simulink model "pitch_control_loop"  (R2025a)
settings: Solver=ode4  StartTime=0.0  StopTime=10.0  FixedStep=0.05  RelTol=1e-3
undefined symbols (not defined in the file or in its folder): pid_damping_b, pitch_inertia
settings Model: Creator=saipr  LastModifiedBy=saipr
settings OptimizationCC: DefaultParameterBehavior=Inlined  EnhancedBackFolding=on  PassReuseOutputArgsAs=Individual arguments  ZeroExternalMemoryAtStartup=off  ZeroInternalMemoryAtStartup=off  OptimizeBlockOrder=speed  DifferentSizesBufferReuse=on  OptimizationCustomize=off  EfficientTunableParamExpr=on
settings DebuggingCC: ParameterTunabilityLossMsg=error
settings SFSimCC: MATLABDynamicMemAlloc=off
settings RTWCC: SystemTargetFile=ert.tlc  TemplateMakefile=ert_default_tmf  GenerateReport=on  GenerateTraceInfo=on  GenerateTraceReport=on  Description=Embedded Coder
settings CodeAppCC: ForceParamTrailComments=on  IgnoreCustomStorageClasses=off  OperatorAnnotations=on  SimulinkDataObjDesc=on  SFDataObjDesc=on  InsertBlockDesc=on
settings ERTTargetCC: ExtModeTransport=0.0  ExtModeStaticAlloc=off  ExtModeMexFile=ext_comm  ExtModeIntrfLevel=Level1  ERTCustomFileTemplate=example_file_process.tlc  TargetLangStandard=C99 (ISO)  GenerateSampleERTMain=on  SupportContinuousTime=on

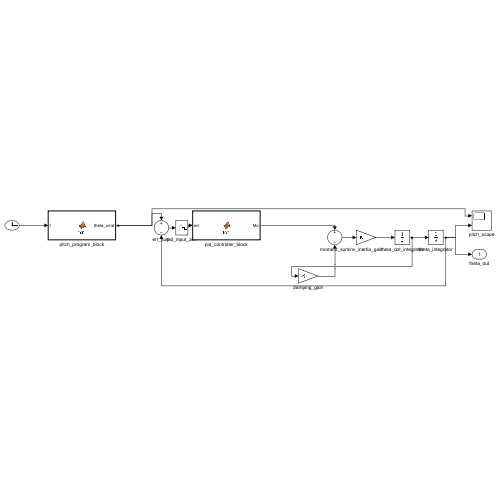
[thumbnail: Simulink's stored preview of the top-level diagram]
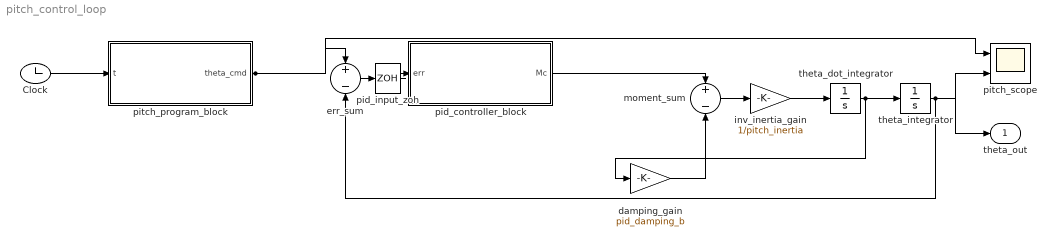
== system pitch_control_loop ==
  Clock : Clock
  damping_gain : Gain  Gain=pid_damping_b
  err_sum : Sum  Inputs=+-
  inv_inertia_gain : Gain  Gain=1/pitch_inertia
  moment_sum : Sum  Inputs=+-
  pid_controller_block : MATLAB Function  TreatAsAtomicUnit=on
  pid_input_zoh : ZeroOrderHold  SampleTime=0.05
  pitch_program_block : MATLAB Function  TreatAsAtomicUnit=on
  pitch_scope : Scope  NumInputPorts=2
  theta_dot_integrator : Integrator
  theta_integrator : Integrator
  theta_out : Outport
  wires:
  Clock/1 -> pitch_program_block/1(t)
  pitch_program_block/1(theta_cmd) -> err_sum/1, pitch_scope/1
  err_sum/1 -> pid_input_zoh/1
  pid_input_zoh/1 -> pid_controller_block/1(err)
  pid_controller_block/1(Mc) -> moment_sum/1
  theta_dot_integrator/1 -> damping_gain/1, theta_integrator/1
  damping_gain/1 -> moment_sum/2
  moment_sum/1 -> inv_inertia_gain/1
  inv_inertia_gain/1 -> theta_dot_integrator/1
  theta_integrator/1 -> err_sum/2, theta_out/1, pitch_scope/2

== matlab function pitch_control_loop/pitch_program_block ==
  data: t input; theta_cmd output
function theta_cmd = pitch_program_block(t)
% Embedded Coder-compatible port of src/guidance/pitch_program.m.
% Constants inlined (MATLAB Function blocks do not accept struct
% inputs from config/*.m directly without extra setup); keep in
% sync with config/simulation_settings.m ss.pitch fields by hand,
% documented in docs/01_design_decisions.md.
t_vertical = 10.0; t_kick_end = 15.0; kick_deg = 3.0;
t_pitch_end = 260.0; theta_final_deg = 6.0;
if t < t_vertical
    theta_cmd_deg = 90.0;
elseif t < t_kick_end
    frac = (t - t_vertical) / (t_kick_end - t_vertical);
    theta_cmd_deg = 90.0 - kick_deg * frac;
else
    theta_kick = 90.0 - kick_deg;
    if t < t_pitch_end
        frac = (t - t_kick_end) / (t_pitch_end - t_kick_end);
        theta_cmd_deg = theta_kick + (theta_final_deg - theta_kick) * frac;
    else
        theta_cmd_deg = theta_final_deg;
    end
end
theta_cmd = theta_cmd_deg * pi / 180;

== matlab function pitch_control_loop/pid_controller_block ==
  data: err input; Mc output
function Mc = pid_controller_block(err)
% Embedded Coder-compatible port of src/control/pid_update.m,
% using persistent variables for controller state (the idiomatic
% Simulink/Embedded-Coder pattern) instead of the explicit
% struct-in/struct-out signature used in the plain-MATLAB
% version -- structs crossing a MATLAB Function block boundary
% need extra bus/type setup that is not worth the complexity
% here. Gains are inlined; keep in sync with
% config/vehicle_parameters.m vp.pid by hand.
persistent integral prev_err first_call
if isempty(first_call)
    integral = 0.0; prev_err = 0.0; first_call = true;
end
kp = 800000.0; ki = 5000.0; kd = 250000.0; out_limit = 2.0e6;
dt = 0.05;
integral = integral + err * dt;
if first_call
    deriv = 0.0;
else
    deriv = (err - prev_err) / dt;
end
u_unsat = kp*err + ki*integral + kd*deriv;
Mc = max(min(u_unsat, out_limit), -out_limit);
prev_err = err;
first_call = false;
